simulink model "Primeira_lei_de_controle (1)"  (R2015b)
settings: Solver=VariableStepAuto  StartTime=0.0  StopTime=10.0  RelTol=1e-3
settings Model: Creator=egidio.neto  LastModifiedBy=egidio.neto

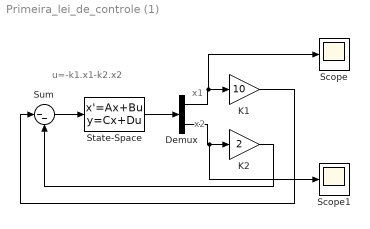
== system Primeira_lei_de_controle (1) ==
  note: x2
  note: x1
  note: u=-k1.x1-k2.x2
  Demux : Demux  Outputs=2
  K1 : Gain  Gain=10
  K2 : Gain  Gain=2
  Scope : Scope
  Scope1 : Scope
  State-Space : StateSpace  A=[0 1; -1 -2]  B=[0;1]  C=[1 0; 0 1]  D=[0;0]  X0=[0.5; 0]
  Sum : Sum  Inputs=|--
  wires:
  State-Space/1 -> Demux/1
  Demux/1 -> Scope/1, K1/1
  Demux/2 -> Scope1/1, K2/1
  Sum/1 -> State-Space/1
  K2/1 -> Sum/2
  K1/1 -> Sum/1
